simulink model "MME321_Lab5_Simulink"  (R2024a)
settings: Solver=VariableStepAuto  StartTime=0.0  StopTime=60  RelTol=1e-3
undefined symbols (not defined in the file): B, J, Ke, Kt, L, R, V
settings Model: Creator=buttrakd  LastModifiedBy=buttrakd

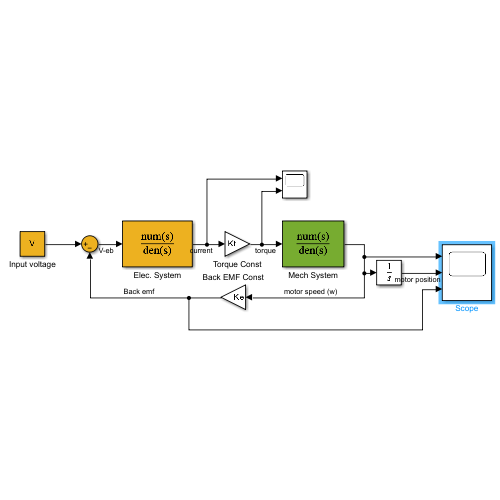
[thumbnail: Simulink's stored preview of the top-level diagram]
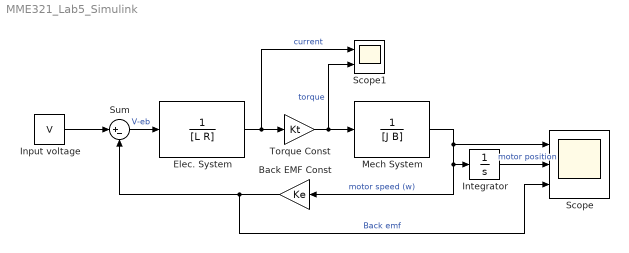
== system MME321_Lab5_Simulink ==
  Back EMF Const : Gain  Gain=Ke
  Elec. System : TransferFcn  Denominator=[L R]
  Input voltage : Constant  Value=V
  Integrator : Integrator
  Mech System : TransferFcn  Denominator=[J B]
  Scope : Scope  NumInputPorts=3
  Scope1 : Scope  NumInputPorts=2
  Sum : Sum  Inputs=|+-
  Torque Const : Gain  Gain=Kt
  wires:
  Sum/1 -> Elec. System/1  "V-eb"
  Elec. System/1 -> Scope1/1, Torque Const/1  "current"
  Torque Const/1 -> Scope1/2, Mech System/1  "torque"
  Mech System/1 -> Integrator/1, Back EMF Const/1, Scope/1  "motor speed (w)"
  Back EMF Const/1 -> Scope/3, Sum/2  "Back emf"
  Input voltage/1 -> Sum/1
  Integrator/1 -> Scope/2  "motor position"
